simulink model "servo_motor"  (R2024a)
settings: Solver=ode15s  StartTime=0.0  StopTime=5.0  RelTol=1e-3
model workspace (MAT data in the model file):
  J = 5e-05
  K = 0.2
  L = 0.01
  R = 4
  Ts = 0.01
  V = 7.4
  b = 0.0005
  ki = 7.33
  kp = 9.39
settings Model: Creator=nacer  LastModifiedBy=nacer
settings SolverCC: AlgebraicLoopSolver=TrustRegion
settings DataIOCC: ReturnWorkspaceOutputs=off
settings DebuggingCC: UnconnectedInputMsg=warning  UnconnectedOutputMsg=warning  UnconnectedLineMsg=warning  ArithmeticOperatorsInVariantConditions=warning
settings ModelReferenceCC: EnableRefExpFcnMdlSchedulingChecks=on
settings SFSimCC: CustomCodeUndefinedFunction=UseInterfaceOnly
settings RTWCC: GPUComputeCapability=3.5

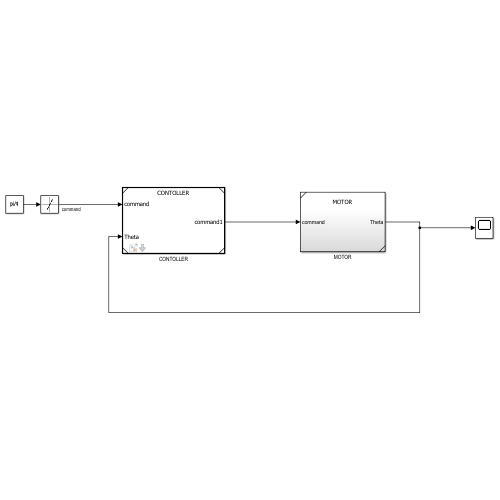
[thumbnail: Simulink's stored preview of the top-level diagram]
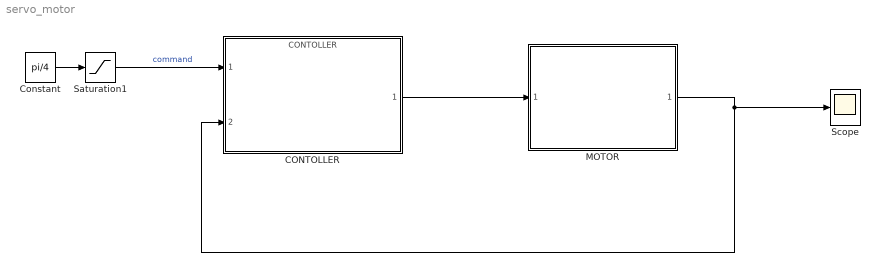
== system servo_motor ==
  CONTOLLER : ModelReference  ModelNameDialog=CONTOLLER  UsingDefaultArgumentValue=0,0,0  SimulationMode=Normal  ModelReferenceVersion=12.5  Ts=0.01  ki=7.33  kp=9.39
  Constant : Constant  Value=pi/4
  MOTOR : Subsystem  ReferencedSubsystem=MOTOR
  Saturation1 : Saturate  UpperLimit=pi/4  LowerLimit=-pi/4
  Scope : Scope
  wires:
  Constant/1 -> Saturation1/1
  MOTOR/1 -> CONTOLLER/2, Scope/1
  Saturation1/1 -> CONTOLLER/1  "command"
  CONTOLLER/1 -> MOTOR/1
